simulink model "s0432"  (Simulink 7.0)
settings: Solver=ode3  SolverMode=SingleTasking  StartTime=0.0  StopTime=900  FixedStep=1  MaxStep=1  RelTol=1e-3  AbsTol=1e-6
values from neighbouring files (symbols this model uses):
  Kpr = 10    [m0108d.m]    (also in m0109b.m = 1; m0113c.m; m0404Bsp.m = 3)
  t0A = -1    [m0404Bsp.m]
undefined symbols (not defined in the file or in its folder): edach, Tr, xD
settings Model: Creator=froriep  LastModifiedBy=froriep
settings DataIOCC: LimitDataPoints=off  SaveOutput=off  SaveTime=off
settings OptimizationCC: BooleanDataType=off
settings DebuggingCC: SaveWithParameterizedLinksMsg=none  SignalResolutionControl=TryResolveAllWithWarning  SolverPrmCheckMsg=none  MultiTaskDSMMsg=warning  MultiTaskCondExecSysMsg=none  StrictBusMsg=None
settings HardwareCC: TargetUnknown=on
settings RTWCC: IncludeERTFirstTime=on

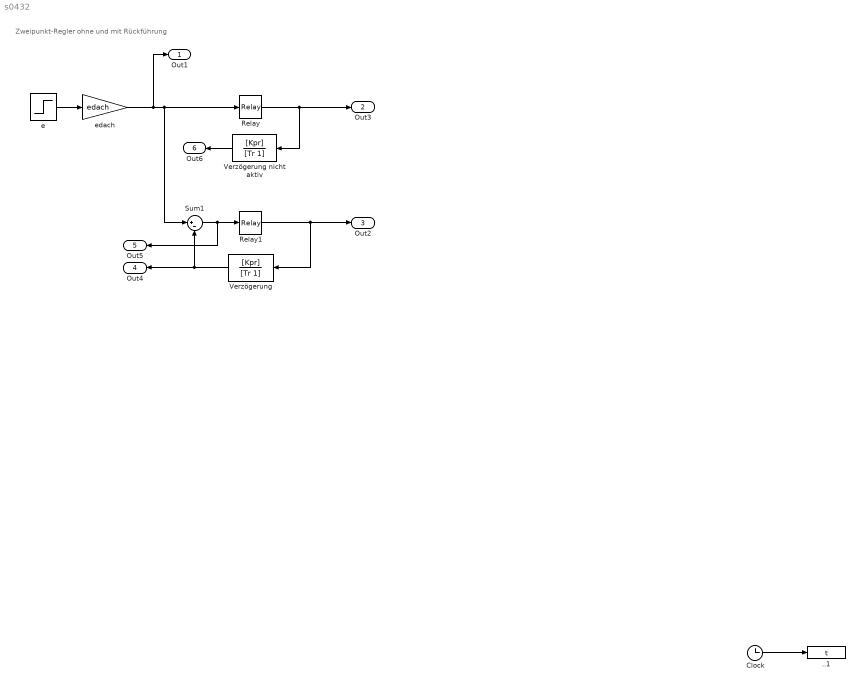
== system s0432 ==
  note: Zweipunkt-Regler ohne und mit Rückführung
  ..1 : ToWorkspace  VariableName=t  SaveFormat=Array
  Clock : Clock
      settings: Decimation=10
  Relay : Relay  OnSwitchValue=xD/2  OffSwitchValue=-xD/2  OnOutputValue=Yh  OutDataType=sfix(16)  OutScaling=2^0
  Relay1 : Relay  OnSwitchValue=xD/2  OffSwitchValue=-xD/2  OnOutputValue=Yh  OutDataType=sfix(16)  OutScaling=2^0
  Sum1 : Sum  Inputs=|+-  SaturateOnIntegerOverflow=on  InputSameDT=on
  Verzögerung : TransferFcn  Orientation=left  Numerator=[Kpr]  Denominator=[Tr 1]
  Verzögerung nicht aktiv : TransferFcn  Orientation=left  Numerator=[Kpr]  Denominator=[Tr 1]
  e : Step  Time=-t0A  SampleTime=0
  edach : Gain  Gain=edach  ParameterDataType=sfix(16)  ParameterScaling=2^0  OutDataType=sfix(16)  OutScaling=2^0
  Out1 : Outport  OutDataType=sfix(16)  OutScaling=2^0
  Out3 : Outport  Port=2  OutDataType=sfix(16)  OutScaling=2^0
  Out2 : Outport  Port=3  OutDataType=sfix(16)  OutScaling=2^0
  Out4 : Outport  Orientation=left  Port=4  OutDataType=sfix(16)  OutScaling=2^0
  Out5 : Outport  Orientation=left  Port=5  OutDataType=sfix(16)  OutScaling=2^0
  Out6 : Outport  Orientation=left  Port=6  OutDataType=sfix(16)  OutScaling=2^0
  wires:
  e/1 -> edach/1
  Clock/1 -> ..1/1
  edach/1 -> Out1/1, Relay/1, Sum1/1
  Relay/1 -> Out3/1, Verzögerung nicht aktiv/1
  Sum1/1 -> Relay1/1, Out5/1
  Verzögerung/1 -> Sum1/2, Out4/1
  Relay1/1 -> Verzögerung/1, Out2/1
  Verzögerung nicht aktiv/1 -> Out6/1
